simulink model "output_bin_generate"  (R2024a)
settings: Solver=VariableStepAuto  StartTime=0.0  StopTime=0.1  RelTol=1e-3
values from neighbouring files (symbols this model uses):
  Ts = 1/Fs    (= 7.50007500075e-06)    [new_generation_coeff.m]    (also in simon_test.m; simple_fft_test.m = 1/F; testPSD_c2d.m; testPSD_simulink.m)
libraries: hdlsllib x32
settings Model: Creator=Simon  LastModifiedBy=Simon

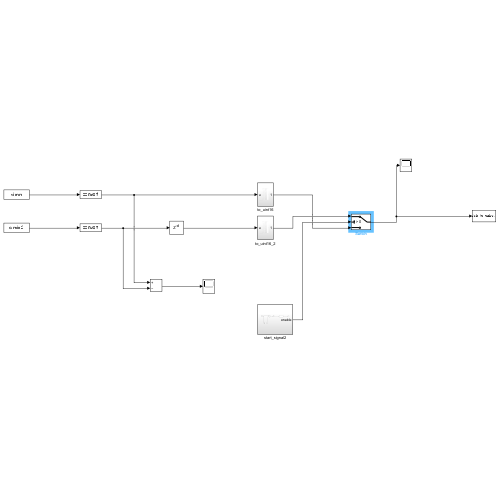
[thumbnail: Simulink's stored preview of the top-level diagram]
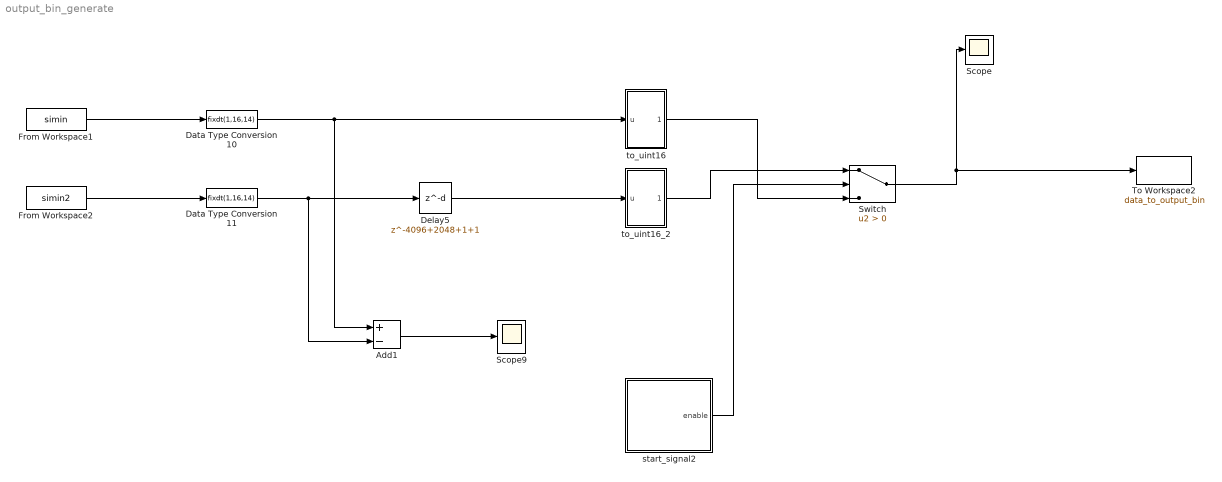
== system output_bin_generate ==
  Add1 : Sum  Inputs=+-
  Data Type Conversion10 : DataTypeConversion  OutDataTypeStr=fixdt(1,16,14)  SaturateOnIntegerOverflow=off  RndMeth=Floor
  Data Type Conversion11 : DataTypeConversion  OutDataTypeStr=fixdt(1,16,14)  SaturateOnIntegerOverflow=off  RndMeth=Floor
  Delay5 : Delay  DelayLength=4096+2048+1+1  InitialCondition=0  SampleTime=Ts
  From Workspace1 : FromWorkspace  VariableName=simin  SampleTime=Ts
  From Workspace2 : FromWorkspace  VariableName=simin2  SampleTime=Ts
  Scope : Scope
  Scope9 : Scope
  Switch : Switch  Criteria=u2 > Threshold  SaturateOnIntegerOverflow=off  InputSameDT=off  OutDataTypeStr=Inherit: Same as first input
  To Workspace2 : ToWorkspace  VariableName=data_to_output_bin  SampleTime=Ts
  start_signal2 : Subsystem
  to_uint16 : Subsystem
  to_uint16_2 : Subsystem
  wires:
  From Workspace2/1 -> Data Type Conversion11/1
  Add1/1 -> Scope9/1
  start_signal2/1(enable) -> Switch/2
  Data Type Conversion11/1 -> Delay5/1, Add1/2
  Data Type Conversion10/1 -> Add1/1, to_uint16/1(u)
  to_uint16_2/1(Out1) -> Switch/1
  From Workspace1/1 -> Data Type Conversion10/1
  Delay5/1 -> to_uint16_2/1(u)
  to_uint16/1(Out1) -> Switch/3
  Switch/1 -> Scope/1, To Workspace2/1

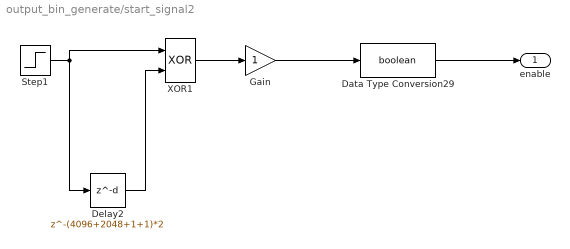
== system output_bin_generate/start_signal2 ==
  Data Type Conversion29 : DataTypeConversion  OutDataTypeStr=boolean  SaturateOnIntegerOverflow=off  RndMeth=Floor
  Delay2 : Delay  DelayLength=(4096+2048+1+1)*2  InitialCondition=0  SampleTime=Ts
  Gain : Gain
  Step1 : Step  Time=Ts*(4096+2048+1+1)  SampleTime=Ts
  XOR1 : Logic  Operator=XOR  IconShape=distinctive  AllPortsSameDT=off  OutDataTypeStr=boolean
  enable : Outport
  wires:
  XOR1/1 -> Gain/1
  Step1/1 -> Delay2/1, XOR1/1
  Delay2/1 -> XOR1/2
  Gain/1 -> Data Type Conversion29/1
  Data Type Conversion29/1 -> enable/1

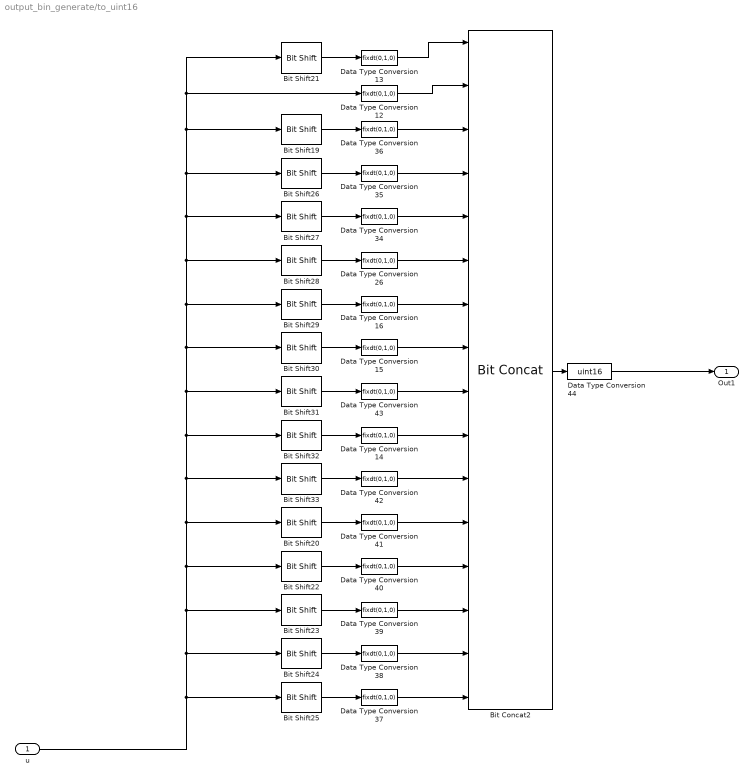
== system output_bin_generate/to_uint16 ==
  u : Inport
  Bit Concat2 : hdlsllib/Logic and Bit Operations/Bit Concat  numInputs=16
  Bit Shift19 : hdlsllib/Logic and Bit Operations/Bit Shift  mode=Shift Left Logical  N=1
  Bit Shift20 : hdlsllib/Logic and Bit Operations/Bit Shift  mode=Shift Left Logical  N=10
  Bit Shift21 : hdlsllib/Logic and Bit Operations/Bit Shift  mode=Shift Right Logical  N=1
  Bit Shift22 : hdlsllib/Logic and Bit Operations/Bit Shift  mode=Shift Left Logical  N=11
  Bit Shift23 : hdlsllib/Logic and Bit Operations/Bit Shift  mode=Shift Left Logical  N=12
  Bit Shift24 : hdlsllib/Logic and Bit Operations/Bit Shift  mode=Shift Left Logical  N=13
  Bit Shift25 : hdlsllib/Logic and Bit Operations/Bit Shift  mode=Shift Left Logical  N=14
  Bit Shift26 : hdlsllib/Logic and Bit Operations/Bit Shift  mode=Shift Left Logical  N=2
  Bit Shift27 : hdlsllib/Logic and Bit Operations/Bit Shift  mode=Shift Left Logical  N=3
  Bit Shift28 : hdlsllib/Logic and Bit Operations/Bit Shift  mode=Shift Left Logical  N=4
  Bit Shift29 : hdlsllib/Logic and Bit Operations/Bit Shift  mode=Shift Left Logical  N=5
  Bit Shift30 : hdlsllib/Logic and Bit Operations/Bit Shift  mode=Shift Left Logical  N=6
  Bit Shift31 : hdlsllib/Logic and Bit Operations/Bit Shift  mode=Shift Left Logical  N=7
  Bit Shift32 : hdlsllib/Logic and Bit Operations/Bit Shift  mode=Shift Left Logical  N=8
  Bit Shift33 : hdlsllib/Logic and Bit Operations/Bit Shift  mode=Shift Left Logical  N=9
  Data Type Conversion{12..16,26,34..43} (16 alike) : DataTypeConversion  OutDataTypeStr=fixdt(0,1,0)  SaturateOnIntegerOverflow=off  RndMeth=Floor
  Data Type Conversion44 : DataTypeConversion  OutDataTypeStr=uint16  SaturateOnIntegerOverflow=off  RndMeth=Floor
  Out1 : Outport
  wires:
  Bit Shift22/1 -> Data Type Conversion40/1
  Bit Shift27/1 -> Data Type Conversion34/1
  Data Type Conversion36/1 -> Bit Concat2/3
  u/1 -> Bit Shift21/1, Data Type Conversion12/1, Bit Shift19/1, Bit Shift26/1, Bit Shift27/1, Bit Shift28/1, Bit Shift29/1, Bit Shift30/1, Bit Shift31/1, Bit Shift32/1, Bit Shift33/1, Bit Shift20/1, Bit Shift22/1, Bit Shift23/1, Bit Shift24/1, Bit Shift25/1
  Bit Shift20/1 -> Data Type Conversion41/1
  Data Type Conversion13/1 -> Bit Concat2/1
  Data Type Conversion40/1 -> Bit Concat2/13
  Bit Shift31/1 -> Data Type Conversion43/1
  Data Type Conversion26/1 -> Bit Concat2/6
  Data Type Conversion44/1 -> Out1/1
  Data Type Conversion35/1 -> Bit Concat2/4
  Data Type Conversion42/1 -> Bit Concat2/11
  Bit Shift19/1 -> Data Type Conversion36/1
  Data Type Conversion38/1 -> Bit Concat2/15
  Bit Shift25/1 -> Data Type Conversion37/1
  Data Type Conversion15/1 -> Bit Concat2/8
  Bit Shift30/1 -> Data Type Conversion15/1
  Data Type Conversion12/1 -> Bit Concat2/2
  Bit Shift32/1 -> Data Type Conversion14/1
  Data Type Conversion39/1 -> Bit Concat2/14
  Data Type Conversion34/1 -> Bit Concat2/5
  Data Type Conversion43/1 -> Bit Concat2/9
  Data Type Conversion16/1 -> Bit Concat2/7
  Bit Shift33/1 -> Data Type Conversion42/1
  Bit Shift24/1 -> Data Type Conversion38/1
  Data Type Conversion41/1 -> Bit Concat2/12
  Bit Shift23/1 -> Data Type Conversion39/1
  Bit Shift29/1 -> Data Type Conversion16/1
  Data Type Conversion37/1 -> Bit Concat2/16
  Bit Shift28/1 -> Data Type Conversion26/1
  Bit Shift21/1 -> Data Type Conversion13/1
  Bit Shift26/1 -> Data Type Conversion35/1
  Bit Concat2/1 -> Data Type Conversion44/1
  Data Type Conversion14/1 -> Bit Concat2/10

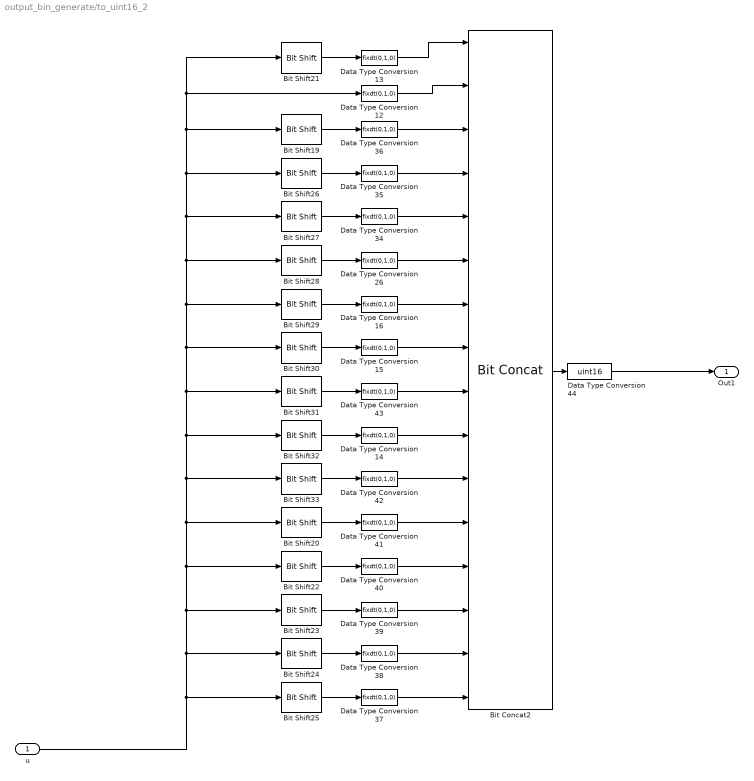
== system output_bin_generate/to_uint16_2 ==
  u : Inport
  Bit Concat2 : hdlsllib/Logic and Bit Operations/Bit Concat  numInputs=16
  Bit Shift19 : hdlsllib/Logic and Bit Operations/Bit Shift  mode=Shift Left Logical  N=1
  Bit Shift20 : hdlsllib/Logic and Bit Operations/Bit Shift  mode=Shift Left Logical  N=10
  Bit Shift21 : hdlsllib/Logic and Bit Operations/Bit Shift  mode=Shift Right Logical  N=1
  Bit Shift22 : hdlsllib/Logic and Bit Operations/Bit Shift  mode=Shift Left Logical  N=11
  Bit Shift23 : hdlsllib/Logic and Bit Operations/Bit Shift  mode=Shift Left Logical  N=12
  Bit Shift24 : hdlsllib/Logic and Bit Operations/Bit Shift  mode=Shift Left Logical  N=13
  Bit Shift25 : hdlsllib/Logic and Bit Operations/Bit Shift  mode=Shift Left Logical  N=14
  Bit Shift26 : hdlsllib/Logic and Bit Operations/Bit Shift  mode=Shift Left Logical  N=2
  Bit Shift27 : hdlsllib/Logic and Bit Operations/Bit Shift  mode=Shift Left Logical  N=3
  Bit Shift28 : hdlsllib/Logic and Bit Operations/Bit Shift  mode=Shift Left Logical  N=4
  Bit Shift29 : hdlsllib/Logic and Bit Operations/Bit Shift  mode=Shift Left Logical  N=5
  Bit Shift30 : hdlsllib/Logic and Bit Operations/Bit Shift  mode=Shift Left Logical  N=6
  Bit Shift31 : hdlsllib/Logic and Bit Operations/Bit Shift  mode=Shift Left Logical  N=7
  Bit Shift32 : hdlsllib/Logic and Bit Operations/Bit Shift  mode=Shift Left Logical  N=8
  Bit Shift33 : hdlsllib/Logic and Bit Operations/Bit Shift  mode=Shift Left Logical  N=9
  Data Type Conversion{12..16,26,34..43} (16 alike) : DataTypeConversion  OutDataTypeStr=fixdt(0,1,0)  SaturateOnIntegerOverflow=off  RndMeth=Floor
  Data Type Conversion44 : DataTypeConversion  OutDataTypeStr=uint16  SaturateOnIntegerOverflow=off  RndMeth=Floor
  Out1 : Outport
  wires:
  Data Type Conversion14/1 -> Bit Concat2/10
  Bit Concat2/1 -> Data Type Conversion44/1
  Bit Shift26/1 -> Data Type Conversion35/1
  Bit Shift21/1 -> Data Type Conversion13/1
  Bit Shift28/1 -> Data Type Conversion26/1
  Data Type Conversion37/1 -> Bit Concat2/16
  Bit Shift29/1 -> Data Type Conversion16/1
  Bit Shift23/1 -> Data Type Conversion39/1
  Data Type Conversion41/1 -> Bit Concat2/12
  Bit Shift24/1 -> Data Type Conversion38/1
  Bit Shift33/1 -> Data Type Conversion42/1
  Data Type Conversion16/1 -> Bit Concat2/7
  Data Type Conversion43/1 -> Bit Concat2/9
  Data Type Conversion34/1 -> Bit Concat2/5
  Data Type Conversion39/1 -> Bit Concat2/14
  Bit Shift32/1 -> Data Type Conversion14/1
  Data Type Conversion12/1 -> Bit Concat2/2
  Bit Shift30/1 -> Data Type Conversion15/1
  Data Type Conversion15/1 -> Bit Concat2/8
  Bit Shift25/1 -> Data Type Conversion37/1
  Data Type Conversion38/1 -> Bit Concat2/15
  Bit Shift19/1 -> Data Type Conversion36/1
  Data Type Conversion42/1 -> Bit Concat2/11
  Data Type Conversion35/1 -> Bit Concat2/4
  Data Type Conversion44/1 -> Out1/1
  Data Type Conversion26/1 -> Bit Concat2/6
  Bit Shift31/1 -> Data Type Conversion43/1
  Data Type Conversion40/1 -> Bit Concat2/13
  Data Type Conversion13/1 -> Bit Concat2/1
  Bit Shift20/1 -> Data Type Conversion41/1
  u/1 -> Bit Shift25/1, Bit Shift24/1, Bit Shift23/1, Bit Shift22/1, Bit Shift20/1, Bit Shift33/1, Bit Shift32/1, Bit Shift31/1, Bit Shift30/1, Bit Shift29/1, Bit Shift28/1, Bit Shift27/1, Bit Shift26/1, Bit Shift19/1, Data Type Conversion12/1, Bit Shift21/1
  Data Type Conversion36/1 -> Bit Concat2/3
  Bit Shift27/1 -> Data Type Conversion34/1
  Bit Shift22/1 -> Data Type Conversion40/1
